simulink model "test"  (R2021a)
settings: Solver=VariableStepAuto  StartTime=0.0  StopTime=10.0  RelTol=1e-3
undefined symbols (not defined in the file): J, Kd
settings Model: Creator=alamg  LastModifiedBy=alamg

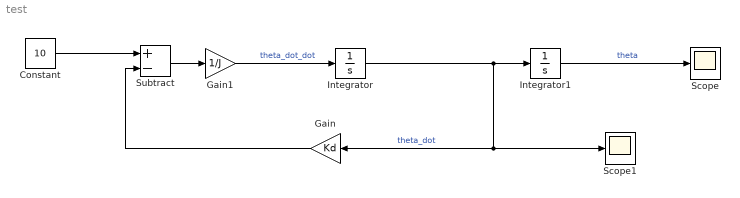
== system test ==
  Constant : Constant  Value=10
  Gain : Gain  Gain=Kd
  Gain1 : Gain  Gain=1/J
  Integrator : Integrator
  Integrator1 : Integrator
  Scope : Scope
  Scope1 : Scope
  Subtract : Sum  Inputs=+-
  wires:
  Integrator/1 -> Scope1/1, Gain/1, Integrator1/1  "theta_dot"
  Gain1/1 -> Integrator/1  "theta_dot_dot"
  Integrator1/1 -> Scope/1  "theta"
  Constant/1 -> Subtract/1
  Gain/1 -> Subtract/2
  Subtract/1 -> Gain1/1
